simulink model "SF011A_EotLrng"  (R2013b)
settings: Solver=FixedStepDiscrete  SolverMode=SingleTasking  StartTime=0.0  StopTime=1  FixedStep=0.002  RelTol=1e-3
values from neighbouring files (symbols this model uses):
  ARCHGLBPRM_FLOATZEROTHD_ULS_F32 = DataDict.Constant    [SF011A_EotLrng_DataDict.m]
  CNVTOMILLISEC_MILLISECPERCNT_F32 = DataDict.Constant    [SF011A_EotLrng_DataDict.m]
  CORRLNFLT_CNT_U08 = DataDict.Constant    [SF011A_EotLrng_DataDict.m]
  DEBSTEP_CNT_U16 = DataDict.Constant    [SF011A_EotLrng_DataDict.m]
  EOTLIMDETD_CNT_LOGL = DataDict.Constant    [SF011A_EotLrng_DataDict.m]
  EOTLIMNOTDETD_CNT_LOGL = DataDict.Constant    [SF011A_EotLrng_DataDict.m]
  EotLrngAuthyStrtLrn = DataDict.Calibration    [SF011A_EotLrng_DataDict.m]
  EotLrngEotLrnTmr = DataDict.Calibration    [SF011A_EotLrng_DataDict.m]
  EotLrngHwAgOverTrvlCnt = DataDict.Calibration    [SF011A_EotLrng_DataDict.m]
  EotLrngHwAgOverTrvlEntr = DataDict.Calibration    [SF011A_EotLrng_DataDict.m]
  EotLrngHwAgOverTrvlExit = DataDict.Calibration    [SF011A_EotLrng_DataDict.m]
  EotLrngHwTqEotLrn = DataDict.Calibration    [SF011A_EotLrng_DataDict.m]
  EotLrngMotVelEotLrn = DataDict.Calibration    [SF011A_EotLrng_DataDict.m]
  EotLrngRackTrvlMax = DataDict.Calibration    [SF011A_EotLrng_DataDict.m]
  EotLrngRackTrvlMin = DataDict.Calibration    [SF011A_EotLrng_DataDict.m]
  EotLrngRstAuthyMin = DataDict.Calibration    [SF011A_EotLrng_DataDict.m]
  EotProtnRackTrvlLimrEna = DataDict.ImprtdCal    [SF011A_EotLrng_DataDict.m]
  HwAgOverTrvl = DataDict.NTC    [SF011A_EotLrng_DataDict.m]
  HWAGOVERTRVLMAXCNT_CNT_U08 = DataDict.Constant    [SF011A_EotLrng_DataDict.m]
  NODEBSTEP_CNT_U16 = DataDict.Constant    [SF011A_EotLrng_DataDict.m]
  OUTOFRNGFLT_CNT_U08 = DataDict.Constant    [SF011A_EotLrng_DataDict.m]
  RackEotStorgFlt = DataDict.NTC    [SF011A_EotLrng_DataDict.m]
  SIGAVLFLT_CNT_U08 = DataDict.Constant    [SF011A_EotLrng_DataDict.m]
undefined symbols (not defined in the file or in its folder): NtcSts1, NvmGetErrSts1, SigQlfr1
libraries: simulink x19, NxtrNvM x12, NxtrAbslt x5, NxtrLim x4, NxtrMax x3, NxtrMin x3
(part 1 of 7)
Description:
  | This function uses vehicle operational information to learn the appropriate end of travel positions for a given system.  Since the position end stop information is important for such functions as
  | end of travel protection to mechanically protect the gear and since the data can vary from one system to the next, it is important to learn these positions
  | 
  | The design also includes features to allow learning to reactivate under conditions of failure or diaganostic service requests (e.g. alignment).
settings Model: PauseTimes=0.35  CovFilter=UTP_SF011A_EotLrng_cov_flt_list  CovHTMLOptions=-sRT=1 -aTS=1 -bRG=1 -bTC=1 -hTR=0 -nFC=0 -scm=1 -bcm=1 -xEv=0  Creator=Mark Kushion  LastModifiedBy=NZ2988
settings SolverCC: AutoInsertRateTranBlk=on  InsertRTBMode=Always
settings DataIOCC: LimitDataPoints=off  SaveFormat=Structure  ReturnWorkspaceOutputs=on
settings OptimizationCC: BlockReduction=off  InlineParams=on  ZeroExternalMemoryAtStartup=off  ZeroInternalMemoryAtStartup=off  OptimizeModelRefInitCode=on  LifeSpan=1
settings DebuggingCC: SignalInfNanChecking=error  SignalRangeChecking=warning  UnderspecifiedInitializationDetection=Simplified  SolverPrmCheckMsg=error  InheritedTsInSrcMsg=error  DiscreteInheritContinuousMsg=error  SingleTaskRateTransMsg=error  TasksWithSamePriorityMsg=error  SigSpecEnsureSampleTimeMsg=error  CheckMatrixSingularityMsg=error  ParameterUnderflowMsg=error  ParameterPrecisionLossMsg=error  ParameterTunabilityLossMsg=error  FixptConstUnderflowMsg=warning  FixptConstOverflowMsg=warning  VectorMatrixConversionMsg=error  SignalLabelMismatchMsg=error  UnconnectedInputMsg=error  UnconnectedOutputMsg=error  UnconnectedLineMsg=error  SFcnCompatibilityMsg=error  UniqueDataStoreMsg=warning  BusObjectLabelMismatch=error  RootOutportRequireBusObject=error  AssertControl=DisableAll  ModelReferenceIOMsg=error  ModelReferenceVersionMismatchMessage=warning  ModelReferenceIOMismatchMessage=error  ModelReferenceCSMismatchMessage=warning  ModelReferenceDataLoggingMessage=error  StateNameClashWarn=warning  StrictBusMsg=ErrorOnBusTreatedAsVector  NonBusSignalsTreatedAsBus=error  SFUnexpectedBacktrackingDiag=error  SFInvalidInputDataAccessInChartInitDiag=error  SFNoUnconditionalDefaultTransitionDiag=error  SFTransitionOutsideNaturalParentDiag=error  SFUnconditionalTransitionShadowingDiag=error  SFUndirectedBroadcastEventsDiag=error
settings ModelReferenceCC: ModelReferenceNumInstancesAllowed=Single
settings RTWCC: SystemTargetFile=autosar.tlc  GenCodeOnly=on  TemplateMakefile=ert_default_tmf  Description=AUTOSAR  GenerateReport=on  ProcessScript=autosar_make_rtw_hook  LaunchReport=on
settings CodeAppCC: GenerateComments=off  IgnoreCustomStorageClasses=off  CustomSymbolStrType=$N$R$M  CustomSymbolStrBlkIO=$N$M  SimulinkBlockComments=off
settings STFCustomTargetCC: ParMdlRefBuildCompliant=on  CompOptLevelCompliant=on  IncludeMdlTerminateFcn=off  CombineOutputUpdateFcns=on  SuppressErrorStatus=on  ERTFirstTimeCompliant=on  ERTCustomFileBanners=on  SupportNonFinite=off  SupportComplex=off  SupportContinuousTime=off  SupportNonInlinedSFcns=off  MATLABClassNameForMDSCustomization=Simulink.SoftwareTarget.ERTCustomization  AutosarCompliant=on  GRTInterface=off  SystemTargetFile=autosar.tlc
settings ERTTargetCC: CodeReplacementLibrary=ANSI_C  ConcurrentExecutionCompliant=off  IncludeMdlTerminateFcn=off  SuppressErrorStatus=on  SupportNonFinite=off  SupportComplex=off  ModelStepFunctionPrototypeControlCompliant=off  CPPClassGenCompliant=off  AutosarCompliant=on  InlinedParameterPlacement=NonHierarchical  ERTCustomFileTemplate=example_file_process.tlc  EnableUserReplacementTypes=on

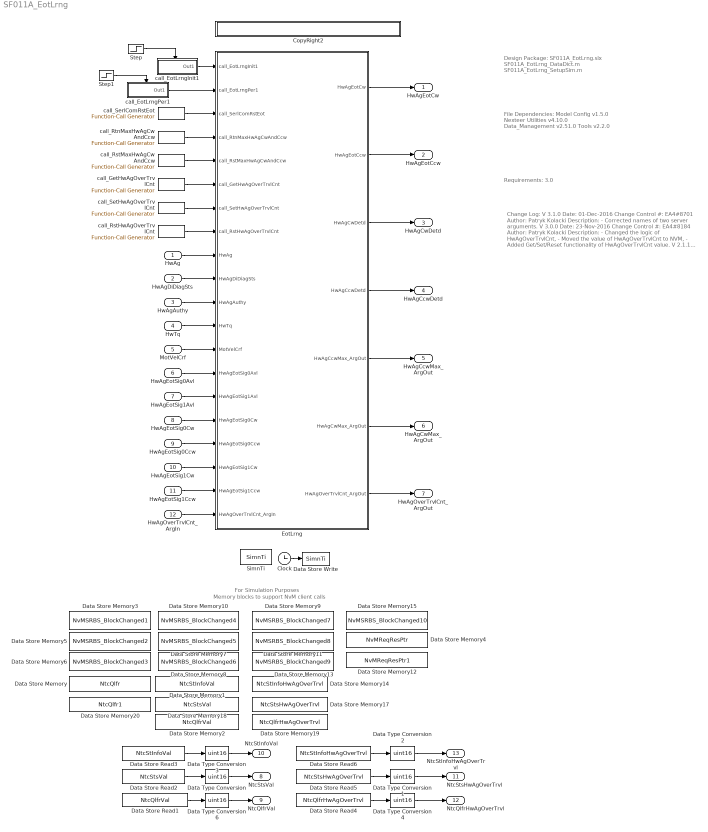
== system SF011A_EotLrng ==
  note: Requirements: 3.0
  note: File Dependencies:
      |
      | Model Config v1.5.0
      | Nexteer Utilities v4.10.0
      | Data_Management v2.51.0
      | Tools v2.2.0
  note: Change Log:
      | V 3.1.0
      | Date: 01-Dec-2016
      | Change Control #: EA4#8701
      | Author: Patryk Kolacki
      | Description:
      | - Corrected names of two server arguments.
      |
      | V 3.0.0
      | Date: 23-Nov-2016
      | Change Control #: EA4#8184
      | Author: Patryk Kolacki
      | Description:
      | - Changed the logic of HwAgOverTrvlCnt,
      | - Moved the value of HwAgOverTrvlCnt to NVM,
      | - Added Get/Set/Reset functionality of HwAgOverTrvlCnt value.
      |
      | V 2.1.1
      | Date: 02-Aug-2016
      | Change Control #: EA4#6725
      | Description:
      | - Changed the NtcQlfr to NtcQlfr1 in NTC blocks of NTC 0x0A7 for simulation
      |   purpose.
      |
      | V 2.1.0
      | Date: 13-Jun-2016
      | Change Control #: EA4#6115
      | Author: Sudeep shankar
      | Description:
      | - "Over travel" diagnostic NTC is set when HW position is outside
      | of  EOT limit.
      | - NTCNR_0X0E1.NtcTyp is changed from 'None' to 'Deb' in
      | DataDictionary for NTCNR_0X0E1 NTC.
      |
      | V 2.0.0
      | Date: 18-May-2016
      | Change Control #: EA4#5532
      | Author: Sudeep shankar
      | Description:
      | - Added logic to determine Max HwAg Cw and Ccw seen by the gear
      | over life of gear
      |
      | V 1.4.0
      | Date: 04-Jan-2016
      | Change Control #: 3583
      | Author: Shailesh Singh/Muragesh(KPIT)
      | Description:
      | - EotNvmData.EngInit changed from struct to []
      | Changed Data Store Memory 7 / Signal Attributes / Initial Value
      | from struct to []
      |
      | V 1.3.0
      | Date: 1-Oct-2015
      | Change Control #: 1216
      | Author: Sudeep Shankar
      | Description:
      | - Nvm and GetRefTmr100MicroSec32bit "Call-Location" updated in DD
      | - RTE write calls for output signals updated in DD
      | - RTE output names for Init1 are aligned with periodic
      | - Added limit blocks in Init to limit outputs
      |
      | V 1.2.0
      | Date: 28-Sep-2015
      | Change Control #: 1216
      | Author: Sudeep Shankar
      | Description:
      | - GetError Status is compared against enum to verify validity of NVM
      | - Init block is added with Min max range check of Eot limits and invoke
      |   reset Eot if out of range
      | - In periodic, Reset Eot block is replaced with the same as used in Init
      |    and updated annotation
      | - Boolean Constant name changed from '_LGC' to '_LOGL' as per
      |   EA4 naming standards
      | - Min Max range check corrected for Ccw inside SRL enable block
      |
      |
      | V1.1.0:
      | Date: 20-Sep-2105
      | Change Control #: 1216
      | Author: Sudeep Shankar
      | Description: Cw and Ccw range update in DataDictonary.
      |
      |
      | V 1.0.0
      | Date: 15-Sep-2015
      | Change Control #: 1216
      | Author: Sudeep Shankar
      | Description:
      | - Initial Release based on EA3 V 6.0.0 and added logic to use learned
      |  limits from control module based on SRL enable.
  note: For Simulation Purposes
  note: Memory blocks to support NvM client calls
  note: Design Package:
      |
      | SF011A_EotLrng.slx
      | SF011A_EotLrng_DataDict.m
      | SF011A_EotLrng_SetupSim.m
  HwAg : Inport
  HwAgDiDiagSts : Inport  Port=2
  HwAgAuthy : Inport  Port=3
  HwTq : Inport  Port=4
  MotVelCrf : Inport  Port=5
  HwAgEotSig0Avl : Inport  RequirementInfo={} %GIDa_73aa7372_5f3f_4a20_9c9f_25262da9d972  Port=6
  HwAgEotSig1Avl : Inport  RequirementInfo={} %GIDa_66c51ce2_8578_4348_9fad_52cccaaeb985  Port=7
  HwAgEotSig0Cw : Inport  RequirementInfo={} %GIDa_a5f7fcd9_8a24_4cbe_b701_71991071193b  Port=8
  HwAgEotSig0Ccw : Inport  RequirementInfo={} %GIDa_9a8ac91a_a1c0_4442_a2c5_4b419678d76d  Port=9
  HwAgEotSig1Cw : Inport  RequirementInfo={} %GIDa_8f8e183e_8cba_4267_90ea_415514e5b391  Port=10
  HwAgEotSig1Ccw : Inport  RequirementInfo={} %GIDa_19e35c30_ed39_4f4a_8321_5e5ce81c406e  Port=11
  HwAgOverTrvlCnt_ArgIn : Inport  RequirementInfo={} %GIDa_de79dbd8_1f60_4db4_9d0d_a8f19dcbcdc4  Port=12
  Clock : Clock
  CopyRight2 : Subsystem  Description=|  mask(Copyright Information){none=on}
      | Copyright info block.                                               
      |                                                                     
      | Place copyright information at the top of every subsystem in design.
      mask prompts: none "No parameters"
      mask help: Place copyright information at the top of every subsystem in design.
      mask Display:
      | NxtrConf = 'Nexteer Confidential';
      | 
      | sys = bdroot; %handle for the current model ("system")
      | first = get_param(sys,'Created');
      | if(isempty(first))
      |     first = datestr(now,'yyyy');
      | else
      |     first = first(end-3:end);  %year is last four digits
      | end
      | 
      | last = get_param(sys,'LastModifiedDate');
      | if isempty(last)
      |     last = datestr(now,'yyyy');
      | else
      |     last = last(end-3:end);
      | end
      | 
      | if strcmp(first,last)
      |     fprintf('%s -- Copyright %s Nexteer',NxtrConf,first)
      | else
      |     fprintf('%s -- %s%s- %s Nexteer',NxtrConf,char(169),first,last)
      | end
  Data Store Memory : DataStoreMemory  DataStoreName=NtcQlfr  InitialValue=SigQlfr1.SIGQLFR_NORES  OutDataTypeStr=Enum: SigQlfr1
  Data Store Memory1 : DataStoreMemory  DataStoreName=NtcStInfoVal  OutDataTypeStr=uint8
  Data Store Memory10 : DataStoreMemory  DataStoreName=NvMSRBS_BlockChanged4  ReadBeforeWriteMsg=warning  WriteAfterWriteMsg=warning  WriteAfterReadMsg=warning
  Data Store Memory11 : DataStoreMemory  DataStoreName=NvMSRBS_BlockChanged8  ReadBeforeWriteMsg=warning  WriteAfterWriteMsg=warning  WriteAfterReadMsg=warning
  Data Store Memory12 : DataStoreMemory  DataStoreName=NvMReqResPtr1
  Data Store Memory13 : DataStoreMemory  DataStoreName=NvMSRBS_BlockChanged9  ReadBeforeWriteMsg=warning  WriteAfterWriteMsg=warning  WriteAfterReadMsg=warning
  Data Store Memory14 : DataStoreMemory  DataStoreName=NtcStInfoHwAgOverTrvl  OutDataTypeStr=uint8
  Data Store Memory15 : DataStoreMemory  DataStoreName=NvMSRBS_BlockChanged10  ReadBeforeWriteMsg=warning  WriteAfterWriteMsg=warning  WriteAfterReadMsg=warning
  Data Store Memory17 : DataStoreMemory  DataStoreName=NtcStsHwAgOverTrvl  InitialValue=NtcSts1.NTCSTS_PASSD  OutDataTypeStr=Enum: NtcSts1
  Data Store Memory18 : DataStoreMemory  DataStoreName=NtcStsVal  InitialValue=NtcSts1.NTCSTS_PASSD  OutDataTypeStr=Enum: NtcSts1
  Data Store Memory19 : DataStoreMemory  DataStoreName=NtcQlfrHwAgOverTrvl  InitialValue=SigQlfr1.SIGQLFR_NORES  OutDataTypeStr=Enum: SigQlfr1
  Data Store Memory2 : DataStoreMemory  DataStoreName=NtcQlfrVal  InitialValue=SigQlfr1.SIGQLFR_NORES  OutDataTypeStr=Enum: SigQlfr1
  Data Store Memory20 : DataStoreMemory  DataStoreName=NtcQlfr1  InitialValue=SigQlfr1.SIGQLFR_NORES  OutDataTypeStr=Enum: SigQlfr1
  Data Store Memory3 : DataStoreMemory  DataStoreName=NvMSRBS_BlockChanged1  ReadBeforeWriteMsg=warning  WriteAfterWriteMsg=warning  WriteAfterReadMsg=warning
  Data Store Memory4 : DataStoreMemory  DataStoreName=NvMReqResPtr
  Data Store Memory5 : DataStoreMemory  DataStoreName=NvMSRBS_BlockChanged2  ReadBeforeWriteMsg=warning  WriteAfterWriteMsg=warning  WriteAfterReadMsg=warning
  Data Store Memory6 : DataStoreMemory  DataStoreName=NvMSRBS_BlockChanged3  ReadBeforeWriteMsg=warning  WriteAfterWriteMsg=warning  WriteAfterReadMsg=warning
  Data Store Memory7 : DataStoreMemory  DataStoreName=NvMSRBS_BlockChanged5  ReadBeforeWriteMsg=warning  WriteAfterWriteMsg=warning  WriteAfterReadMsg=warning
  Data Store Memory8 : DataStoreMemory  DataStoreName=NvMSRBS_BlockChanged6  ReadBeforeWriteMsg=warning  WriteAfterWriteMsg=warning  WriteAfterReadMsg=warning
  Data Store Memory9 : DataStoreMemory  DataStoreName=NvMSRBS_BlockChanged7  ReadBeforeWriteMsg=warning  WriteAfterWriteMsg=warning  WriteAfterReadMsg=warning
  Data Store Read1 : DataStoreRead  DataStoreName=NtcQlfrVal  SampleTime=.010
  Data Store Read2 : DataStoreRead  DataStoreName=NtcStsVal  SampleTime=.010
  Data Store Read3 : DataStoreRead  DataStoreName=NtcStInfoVal  SampleTime=.010
  Data Store Read4 : DataStoreRead  DataStoreName=NtcQlfrHwAgOverTrvl  SampleTime=.010
  Data Store Read5 : DataStoreRead  DataStoreName=NtcStsHwAgOverTrvl  SampleTime=.010
  Data Store Read6 : DataStoreRead  DataStoreName=NtcStInfoHwAgOverTrvl  SampleTime=.010
  Data Store Write : DataStoreWrite  DataStoreName=SimnTi
  Data Type Conversion{,1..4,6} (6 alike) : DataTypeConversion  OutDataTypeStr=uint16
  EotLrng : Subsystem
  SimnTi : DataStoreMemory  DataStoreName=SimnTi
  Step : Step  Time=.001  Before=1  After=0  SampleTime=0
  Step1 : Step  Time=.001  SampleTime=0
  call_EotLrngInit1 : Subsystem  TreatAsAtomicUnit=on
  call_EotLrngPer1 : Subsystem  TreatAsAtomicUnit=on
  call_GetHwAgOverTrvlCnt : simulink/Ports & Subsystems/Function-Call Generator  RequirementInfo={} %GIDa_e3baf494_81de_4b12_b72d_b79894e06156  sample_time=0.010  numberOfIterations=1
  call_RstHwAgOverTrvlCnt : simulink/Ports & Subsystems/Function-Call Generator  RequirementInfo={} %GIDa_03bc3f2a_ba1d_4971_9b17_2c952515d504  sample_time=0.010  numberOfIterations=1
  call_RstMaxHwAgCwAndCcw : simulink/Ports & Subsystems/Function-Call Generator  RequirementInfo={} %GIDa_ce2e9b2d_63af_495d_a1f3_e9201e666fa9  sample_time=0.010  numberOfIterations=1
  call_RtnMaxHwAgCwAndCcw : simulink/Ports & Subsystems/Function-Call Generator  RequirementInfo={} %GIDa_042fcac4_2799_4e4f_8586_b1f6181d77cc  sample_time=0.010  numberOfIterations=1
  call_SerlComRstEot : simulink/Ports & Subsystems/Function-Call Generator  RequirementInfo={} %GIDa_78894832_b76f_4101_86f3_f5347d110ee9  sample_time=0.010  numberOfIterations=1
  call_SetHwAgOverTrvlCnt : simulink/Ports & Subsystems/Function-Call Generator  RequirementInfo={} %GIDa_ec1b0ef1_ec8f_4026_a564_0387bacc0f1d  sample_time=0.010  numberOfIterations=1
  HwAgEotCw : Outport
  HwAgEotCcw : Outport  Port=2
  HwAgCwDetd : Outport  Port=3
  HwAgCcwDetd : Outport  Port=4
  HwAgCcwMax_ArgOut : Outport  Port=5
  HwAgCwMax_ArgOut : Outport  Port=6
  HwAgOverTrvlCnt_ArgOut : Outport  Port=7
  NtcStsVal : Outport  Port=8
  NtcQlfrVal : Outport  Port=9
  NtcStInfoVal : Outport  Port=10
  NtcStsHwAgOverTrvl : Outport  Port=11
  NtcQlfrHwAgOverTrvl : Outport  Port=12
  NtcStInfoHwAgOverTrvl : Outport  Port=13
  wires:
  Clock/1 -> Data Store Write/1
  EotLrng/3(HwAgCwDetd) -> HwAgCwDetd/1
  EotLrng/2(HwAgEotCcw) -> HwAgEotCcw/1
  EotLrng/1(HwAgEotCw) -> HwAgEotCw/1
  EotLrng/4(HwAgCcwDetd) -> HwAgCcwDetd/1
  call_EotLrngInit1/1(Out1) -> EotLrng/1(call_EotLrngInit1)
  Step/1 -> call_EotLrngInit1/Enable
  Step1/1 -> call_EotLrngPer1/Enable
  call_EotLrngPer1/1(Out1) -> EotLrng/2(call_EotLrngPer1)
  call_SerlComRstEot/1 -> EotLrng/3(call_SerlComRstEot)
  Data Store Read1/1 -> Data Type Conversion6/1
  Data Store Read2/1 -> Data Type Conversion/1
  Data Store Read3/1 -> Data Type Conversion3/1
  call_RtnMaxHwAgCwAndCcw/1 -> EotLrng/4(call_RtnMaxHwAgCwAndCcw)
  EotLrng/5(HwAgCcwMax_ArgOut) -> HwAgCcwMax_ArgOut/1
  EotLrng/6(HwAgCwMax_ArgOut) -> HwAgCwMax_ArgOut/1
  call_RstMaxHwAgCwAndCcw/1 -> EotLrng/5(call_RstMaxHwAgCwAndCcw)
  Data Store Read4/1 -> Data Type Conversion4/1
  Data Store Read5/1 -> Data Type Conversion1/1
  Data Store Read6/1 -> Data Type Conversion2/1
  Data Type Conversion2/1 -> NtcStInfoHwAgOverTrvl/1
  Data Type Conversion4/1 -> NtcQlfrHwAgOverTrvl/1
  Data Type Conversion1/1 -> NtcStsHwAgOverTrvl/1
  Data Type Conversion3/1 -> NtcStInfoVal/1
  Data Type Conversion6/1 -> NtcQlfrVal/1
  Data Type Conversion/1 -> NtcStsVal/1
  EotLrng/7(HwAgOverTrvlCnt_ArgOut) -> HwAgOverTrvlCnt_ArgOut/1
  call_GetHwAgOverTrvlCnt/1 -> EotLrng/6(call_GetHwAgOverTrvlCnt)
  call_SetHwAgOverTrvlCnt/1 -> EotLrng/7(call_SetHwAgOverTrvlCnt)
  call_RstHwAgOverTrvlCnt/1 -> EotLrng/8(call_RstHwAgOverTrvlCnt)
  HwAg/1 -> EotLrng/9(HwAg)
  HwAgDiDiagSts/1 -> EotLrng/10(HwAgDiDiagSts)
  HwAgAuthy/1 -> EotLrng/11(HwAgAuthy)
  HwTq/1 -> EotLrng/12(HwTq)
  MotVelCrf/1 -> EotLrng/13(MotVelCrf)
  HwAgEotSig0Avl/1 -> EotLrng/14(HwAgEotSig0Avl)
  HwAgOverTrvlCnt_ArgIn/1 -> EotLrng/20(HwAgOverTrvlCnt_ArgIn)
  HwAgEotSig1Ccw/1 -> EotLrng/19(HwAgEotSig1Ccw)
  HwAgEotSig1Cw/1 -> EotLrng/18(HwAgEotSig1Cw)
  HwAgEotSig0Ccw/1 -> EotLrng/17(HwAgEotSig0Ccw)
  HwAgEotSig0Cw/1 -> EotLrng/16(HwAgEotSig0Cw)
  HwAgEotSig1Avl/1 -> EotLrng/15(HwAgEotSig1Avl)

== system SF011A_EotLrng/CopyRight2 ==

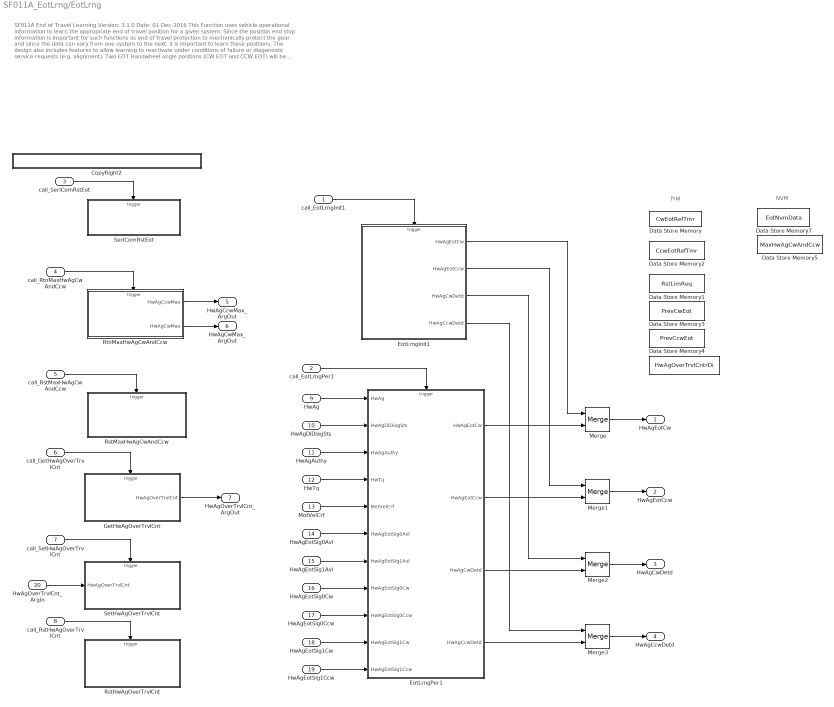
== system SF011A_EotLrng/EotLrng ==
  note: NVM
  note: PIM
  note: SF011A              End of Travel Learning            Version: 3.1.0         Date: 01-Dec-2016
      |
      | This Function uses vehicle operational information to learn the appropriate end of travel position for a given system. Since the position end stop information
      | is important for such functions as end of travel protection to mechanically protect the gear and since the data can vary from one system to the next, it is
      | important to learn these positions.
      |
      | The design also includes features to allow learning to reactivate under conditions of failure or diaganostic service requests (e.g. alignment).
      |
      |  Two EOT Handwheel angle positions (CW EOT and CCW EOT) will be stored in the scratchpad of HW Torque Sensor 0 with a redundant copy  also stored
      |  in the scratchpad of HW Torque Sensor 1 during manufacturing build up. These CW and CCW EOT values will be used for providing the Software Rack
      |  Travel Limits when EotProtnRackTrvlLimrEna is True.
  call_EotLrngInit1 : Inport
  call_EotLrngPer1 : Inport  Port=2
  call_SerlComRstEot : Inport  Port=3
  call_RtnMaxHwAgCwAndCcw : Inport  Port=4
  call_RstMaxHwAgCwAndCcw : Inport  Port=5
  call_GetHwAgOverTrvlCnt : Inport  RequirementInfo={} %GIDa_1cc9e590_aebc_4faa_bf48_c1a914c9f56c  Port=6
  call_SetHwAgOverTrvlCnt : Inport  RequirementInfo={} %GIDa_33957908_3297_46c1_8714_52d5541ebe06  Port=7
  call_RstHwAgOverTrvlCnt : Inport  RequirementInfo={} %GIDa_b35ca6d8_d86b_4ebc_a4ac_db0bdb5da668  Port=8
  HwAg : Inport  RequirementInfo="{'linktype_rmi_doors' '0000ba59 (/E-STEER Core/SubSystem Specifications/Application Functions/SF011A Learned EOT Limits)' '#SF011A_9' 'true' 'REQ:  SF011A_9' '' } %GIDa_42db33ca_01d7_41c2_af64_efb098aee0cd"  Port=9
  HwAgDiDiagSts : Inport  RequirementInfo="{'linktype_rmi_doors' '0000ba59 (/E-STEER Core/SubSystem Specifications/Application Functions/SF011A Learned EOT Limits)' '#SF011A_36' 'true' 'REQ:  SF011A_36' '' } %GIDa_ec3a5a8a_8e2b_48db_b047_1f602cc7cc9a"  Port=10
  HwAgAuthy : Inport  RequirementInfo="{'linktype_rmi_doors' '0000ba59 (/E-STEER Core/SubSystem Specifications/Application Functions/SF011A Learned EOT Limits)' '#SF011A_32' 'true' 'REQ:  SF011A_32' '' } %GIDa_27f0f5a0_b684_4830_bfd2_ef6d05a05c0b"  Port=11
  HwTq : Inport  RequirementInfo="{'linktype_rmi_doors' '0000ba59 (/E-STEER Core/SubSystem Specifications/Application Functions/SF011A Learned EOT Limits)' '#SF011A_34' 'true' 'REQ:  SF011A_34' '' } %GIDa_8b7c6650_fd63_4843_9db1_7f1e52f08757"  Port=12
  MotVelCrf : Inport  RequirementInfo="{'linktype_rmi_doors' '0000ba59 (/E-STEER Core/SubSystem Specifications/Application Functions/SF011A Learned EOT Limits)' '#SF011A_33' 'true' 'REQ:  SF011A_33' '' } %GIDa_72ce3fd6_9cc5_4395_adf3_db347db2b3a0"  Port=13
  HwAgEotSig0Avl : Inport  RequirementInfo="{'linktype_rmi_doors' '0000ba59 (/E-STEER Core/SubSystem Specifications/Application Functions/SF011A Learned EOT Limits)' '#SF011A_116' 'true' 'REQ:  SF011A_116' '' } %GIDa_80459358_5b4f_48e6_a7b8_8da9c9038f81"  Port=14
  HwAgEotSig1Avl : Inport  RequirementInfo="{'linktype_rmi_doors' '0000ba59 (/E-STEER Core/SubSystem Specifications/Application Functions/SF011A Learned EOT Limits)' '#SF011A_116' 'true' 'REQ:  SF011A_116' '' } %GIDa_3caee551_e75b_4d25_be80_97aaac300dbd"  Port=15
  HwAgEotSig0Cw : Inport  RequirementInfo="{'linktype_rmi_doors' '0000ba59 (/E-STEER Core/SubSystem Specifications/Application Functions/SF011A Learned EOT Limits)' '#SF011A_117' 'true' 'REQ:  SF011A_117' '' } %GIDa_c15a533c_6152_4a8a_b933_7aad34b2e7de"  Port=16
  HwAgEotSig0Ccw : Inport  RequirementInfo="{'linktype_rmi_doors' '0000ba59 (/E-STEER Core/SubSystem Specifications/Application Functions/SF011A Learned EOT Limits)' '#SF011A_118' 'true' 'REQ:  SF011A_118' '' } %GIDa_4930c781_ec4f_4ebe_87d2_655a305eb055"  Port=17
  HwAgEotSig1Cw : Inport  RequirementInfo="{'linktype_rmi_doors' '0000ba59 (/E-STEER Core/SubSystem Specifications/Application Functions/SF011A Learned EOT Limits)' '#SF011A_117' 'true' 'REQ:  SF011A_117' '' } %GIDa_5965b097_97b2_4555_a032_94a0a70ed026"  Port=18
  HwAgEotSig1Ccw : Inport  RequirementInfo="{'linktype_rmi_doors' '0000ba59 (/E-STEER Core/SubSystem Specifications/Application Functions/SF011A Learned EOT Limits)' '#SF011A_118' 'true' 'REQ:  SF011A_118' '' } %GIDa_7afbb674_d8de_4557_8f9d_4901633a5dc2"  Port=19
  HwAgOverTrvlCnt_ArgIn : Inport  RequirementInfo="{'linktype_rmi_doors' '0000ba59 (/E-STEER Core/SubSystem Specifications/Application Functions/SF011A Learned EOT Limits)' '#SF011A_201' 'true' 'REQ:  SF011A_201' '' } %GIDa_bf5dc2c4_d885_475e_9768_988ed04b3a3b"  Port=20
  " " : DataStoreMemory  DataStoreName=HwAgOverTrvlCntrDi  StateMustResolveToSignalObject=on
  CopyRight2 : Subsystem  Description=|  mask(Copyright Information){none=on}
      | Copyright info block.                                               
      |                                                                     
      | Place copyright information at the top of every subsystem in design.
      mask prompts: none "No parameters"
      mask help: Place copyright information at the top of every subsystem in design.
      mask Display:
      | NxtrConf = 'Nexteer Confidential';
      | 
      | sys = bdroot; %handle for the current model ("system")
      | first = get_param(sys,'Created');
      | if(isempty(first))
      |     first = datestr(now,'yyyy');
      | else
      |     first = first(end-3:end);  %year is last four digits
      | end
      | 
      | last = get_param(sys,'LastModifiedDate');
      | if isempty(last)
      |     last = datestr(now,'yyyy');
      | else
      |     last = last(end-3:end);
      | end
      | 
      | if strcmp(first,last)
      |     fprintf('%s -- Copyright %s Nexteer',NxtrConf,first)
      | else
      |     fprintf('%s -- %s%s- %s Nexteer',NxtrConf,char(169),first,last)
      | end
  Data Store Memory : DataStoreMemory  DataStoreName=CwEotRefTmr  StateMustResolveToSignalObject=on
  Data Store Memory1 : DataStoreMemory  DataStoreName=RstLimReq  StateMustResolveToSignalObject=on
  Data Store Memory2 : DataStoreMemory  DataStoreName=CcwEotRefTmr  StateMustResolveToSignalObject=on
  Data Store Memory3 : DataStoreMemory  DataStoreName=PrevCwEot  StateMustResolveToSignalObject=on
  Data Store Memory4 : DataStoreMemory  DataStoreName=PrevCcwEot  StateMustResolveToSignalObject=on
  Data Store Memory5 : DataStoreMemory  RequirementInfo="{'linktype_rmi_doors' '0000ba59 (/E-STEER Core/SubSystem Specifications/Application Functions/SF011A Learned EOT Limits)' '#SF011A_209' 'true' 'REQ:  SF011A_209' '' } %GIDa_e44e0bfb_d806_48d4_a199_844757409d5d"  DataStoreName=MaxHwAgCwAndCcw  InitialValue=[]  OutDataTypeStr=Bus: MaxHwAgCwAndCcwRec2  StateMustResolveToSignalObject=on
  Data Store Memory7 : DataStoreMemory  RequirementInfo="{'linktype_rmi_doors' '0000ba59 (/E-STEER Core/SubSystem Specifications/Application Functions/SF011A Learned EOT Limits)' '#SF011A_59' 'true' 'REQ:  SF011A_59' '' ; 'linktype_rmi_doors' '0000ba59 (/E-STEER Core/SubSystem Specifications/Application Functions/SF011A Learned EOT Limits)' '#SF011A_63' 'true' 'REQ:  SF011A_63' '' ; 'linktype_rmi_doors' '0000ba59 (/E-STEER Core/SubSystem Specifications/Application Functions/SF011A Learned EOT Limits)' '#SF011A_62' 'true' 'REQ:  SF011A_62' '' ; 'linktype_rmi_doors' '0000ba59 (/E-STEER Core/SubSystem Specifications/Application Functions/SF011A Learned EOT Limits)' '#SF011A_61' 'true' 'REQ:  SF011A_61' '' ; 'linktype_rmi_doors' '0000ba59 (/E-STEER Core/SubSystem Specifications/Application Functions/SF011A Learned EOT Limits)' '#SF011A_60' 'true' 'REQ:  SF011A_60' '' ; 'linktype_rmi_doors' '0000ba59 (/E-STEER Core/SubSystem Specifications/Application Functions/SF011A Learned EOT Limits)' '#SF011A_111' 'true' 'REQ:  SF011A_111' '' ; 'linktype_rmi_doors' '0000ba59 (/E-STEER Core/SubSystem Specifications/Application Functions/SF011A Learned EOT Limits)' '#SF011A_112' 'true' 'REQ:  SF011A_112' '' ; 'linktype_rmi_doors' '0000ba59 (/E-STEER Core/SubSystem Specifications/Application Functions/SF011A Learned EOT Limits)' '#SF011A_113' 'true' 'REQ:  SF011A_113' '' ; 'linktype_rmi_doors' '0000ba59 (/E-STEER Core/SubSystem Specifications/Application Functions/SF011A Learned EOT Limits)' '#SF011A_114' 'true' 'REQ:  SF011A_114' '' } %GIDa_e5eb2182_a554_401e_b57f_80817cd7d6f2"  DataStoreName=EotNvmData  InitialValue=[]  OutDataTypeStr=Bus: EotNvmDataRec1  StateMustResolveToSignalObject=on
  EotLrngInit1 : Subsystem
  EotLrngPer1 : Subsystem
  GetHwAgOverTrvlCnt : Subsystem  RequirementInfo="{'linktype_rmi_doors' '0000ba59 (/E-STEER Core/SubSystem Specifications/Application Functions/SF011A Learned EOT Limits)' '#SF011A_203' 'true' 'REQ:  SF011A_203' '' } %GIDa_4a5e5f15_a9c8_48fe_986b_cbf465310d0d"
  Merge{,1..3} (4 alike) : Merge
  RstHwAgOverTrvlCnt : Subsystem  RequirementInfo="{'linktype_rmi_doors' '0000ba59 (/E-STEER Core/SubSystem Specifications/Application Functions/SF011A Learned EOT Limits)' '#SF011A_195' 'true' 'REQ:  SF011A_195' '' } %GIDa_9394070d_1ce8_4ba7_93f9_e1140329ccb6"
  RstMaxHwAgCwAndCcw : Subsystem  RequirementInfo="{'linktype_rmi_doors' '0000ba59 (/E-STEER Core/SubSystem Specifications/Application Functions/SF011A Learned EOT Limits)' '#SF011A_160' 'true' 'REQ:  SF011A_160' '' } %GIDa_1fbc0f2a_c98c_4700_a26d_603b800c132e"
  RtnMaxHwAgCwAndCcw : Subsystem  RequirementInfo="{'linktype_rmi_doors' '0000ba59 (/E-STEER Core/SubSystem Specifications/Application Functions/SF011A Learned EOT Limits)' '#SF011A_161' 'true' 'REQ:  SF011A_161' '' } %GIDa_68e311d9_bd4a_4580_880d_d3fc2cfa134d"
  SerlComRstEot : Subsystem  RequirementInfo="{'linktype_rmi_doors' '0000ba59 (/E-STEER Core/SubSystem Specifications/Application Functions/SF011A Learned EOT Limits)' '#SF011A_122' 'true' 'REQ:  SF011A_122' '' } %GIDa_2196a33e_1ec6_460e_afc4_c4580f78035f"
  SetHwAgOverTrvlCnt : Subsystem  RequirementInfo="{'linktype_rmi_doors' '0000ba59 (/E-STEER Core/SubSystem Specifications/Application Functions/SF011A Learned EOT Limits)' '#SF011A_200' 'true' 'REQ:  SF011A_200' '' } %GIDa_51ef5841_6e7a_4466_9fdc_0a858abb14eb"
  HwAgEotCw : Outport  RequirementInfo="{'linktype_rmi_doors' '0000ba59 (/E-STEER Core/SubSystem Specifications/Application Functions/SF011A Learned EOT Limits)' '#SF011A_11' 'true' 'REQ:  SF011A_11' '' } %GIDa_41bb65f1_1f75_476c_89b3_1b3c930dd361"
  HwAgEotCcw : Outport  RequirementInfo="{'linktype_rmi_doors' '0000ba59 (/E-STEER Core/SubSystem Specifications/Application Functions/SF011A Learned EOT Limits)' '#SF011A_39' 'true' 'REQ:  SF011A_39' '' } %GIDa_1bef1b8e_eaa3_4452_9aff_1fc22e093c45"  Port=2
  HwAgCwDetd : Outport  RequirementInfo="{'linktype_rmi_doors' '0000ba59 (/E-STEER Core/SubSystem Specifications/Application Functions/SF011A Learned EOT Limits)' '#SF011A_40' 'true' 'REQ:  SF011A_40' '' } %GIDa_78cdf14d_76bb_44d2_9d5f_dfd0819f21ed"  Port=3
  HwAgCcwDetd : Outport  RequirementInfo="{'linktype_rmi_doors' '0000ba59 (/E-STEER Core/SubSystem Specifications/Application Functions/SF011A Learned EOT Limits)' '#SF011A_41' 'true' 'REQ:  SF011A_41' '' } %GIDa_3fe008c8_2677_4027_a610_4cee2f6e870d"  Port=4
  HwAgCcwMax_ArgOut : Outport  RequirementInfo={} %GIDa_3eec765e_d5a4_4357_9ae4_04adabccafe6  Port=5
  HwAgCwMax_ArgOut : Outport  RequirementInfo={} %GIDa_2634233d_75b1_4c53_9d31_6713fad6f33b  Port=6
  HwAgOverTrvlCnt_ArgOut : Outport  RequirementInfo={} %GIDa_8619cd48_f7b1_49f8_ae7e_1504e94fcefc  Port=7
  wires:
  call_EotLrngPer1/1 -> EotLrngPer1/Trigger
  call_SerlComRstEot/1 -> SerlComRstEot/Trigger
  call_EotLrngInit1/1 -> EotLrngInit1/Trigger
  Merge3/1 -> HwAgCcwDetd/1
  EotLrngPer1/4(HwAgCcwDetd) -> Merge3/2
  EotLrngPer1/3(HwAgCwDetd) -> Merge2/2
  EotLrngPer1/2(HwAgEotCcw) -> Merge1/2
  Merge/1 -> HwAgEotCw/1
  Merge1/1 -> HwAgEotCcw/1
  Merge2/1 -> HwAgCwDetd/1
  EotLrngPer1/1(HwAgEotCw) -> Merge/2
  EotLrngInit1/1(HwAgEotCw) -> Merge/1
  EotLrngInit1/2(HwAgEotCcw) -> Merge1/1
  EotLrngInit1/3(HwAgCwDetd) -> Merge2/1
  EotLrngInit1/4(HwAgCcwDetd) -> Merge3/1
  call_RtnMaxHwAgCwAndCcw/1 -> RtnMaxHwAgCwAndCcw/Trigger
  RtnMaxHwAgCwAndCcw/1(HwAgCcwMax) -> HwAgCcwMax_ArgOut/1
  RtnMaxHwAgCwAndCcw/2(HwAgCwMax) -> HwAgCwMax_ArgOut/1
  call_RstMaxHwAgCwAndCcw/1 -> RstMaxHwAgCwAndCcw/Trigger
  GetHwAgOverTrvlCnt/1(HwAgOverTrvlCnt) -> HwAgOverTrvlCnt_ArgOut/1
  HwAgOverTrvlCnt_ArgIn/1 -> SetHwAgOverTrvlCnt/1(HwAgOverTrvlCnt)
  call_GetHwAgOverTrvlCnt/1 -> GetHwAgOverTrvlCnt/Trigger
  call_SetHwAgOverTrvlCnt/1 -> SetHwAgOverTrvlCnt/Trigger
  call_RstHwAgOverTrvlCnt/1 -> RstHwAgOverTrvlCnt/Trigger
  HwAg/1 -> EotLrngPer1/1(HwAg)
  HwAgDiDiagSts/1 -> EotLrngPer1/2(HwAgDiDiagSts)
  HwAgAuthy/1 -> EotLrngPer1/3(HwAgAuthy)
  HwTq/1 -> EotLrngPer1/4(HwTq)
  MotVelCrf/1 -> EotLrngPer1/5(MotVelCrf)
  HwAgEotSig0Avl/1 -> EotLrngPer1/6(HwAgEotSig0Avl)
  HwAgEotSig1Avl/1 -> EotLrngPer1/7(HwAgEotSig1Avl)
  HwAgEotSig0Cw/1 -> EotLrngPer1/8(HwAgEotSig0Cw)
  HwAgEotSig0Ccw/1 -> EotLrngPer1/9(HwAgEotSig0Ccw)
  HwAgEotSig1Cw/1 -> EotLrngPer1/10(HwAgEotSig1Cw)
  HwAgEotSig1Ccw/1 -> EotLrngPer1/11(HwAgEotSig1Ccw)

== system SF011A_EotLrng/call_EotLrngInit1 ==
  Enable : EnablePort
  CopyRight2 : Subsystem  Description=|  mask(Copyright Information){none=on}
      | Copyright info block.                                               
      |                                                                     
      | Place copyright information at the top of every subsystem in design.
      mask prompts: none "No parameters"
      mask help: Place copyright information at the top of every subsystem in design.
      mask Display:
      | NxtrConf = 'Nexteer Confidential';
      | 
      | sys = bdroot; %handle for the current model ("system")
      | first = get_param(sys,'Created');
      | if(isempty(first))
      |     first = datestr(now,'yyyy');
      | else
      |     first = first(end-3:end);  %year is last four digits
      | end
      | 
      | last = get_param(sys,'LastModifiedDate');
      | if isempty(last)
      |     last = datestr(now,'yyyy');
      | else
      |     last = last(end-3:end);
      | end
      | 
      | if strcmp(first,last)
      |     fprintf('%s -- Copyright %s Nexteer',NxtrConf,first)
      | else
      |     fprintf('%s -- %s%s- %s Nexteer',NxtrConf,char(169),first,last)
      | end
  Function-Call Generator : simulink/Ports & Subsystems/Function-Call Generator  sample_time=.010  numberOfIterations=1
  Out1 : Outport
  wires:
  Function-Call Generator/1 -> Out1/1

== system SF011A_EotLrng/call_EotLrngPer1 ==
  Enable : EnablePort
  CopyRight2 : Subsystem  Description=|  mask(Copyright Information){none=on}
      | Copyright info block.                                               
      |                                                                     
      | Place copyright information at the top of every subsystem in design.
      mask prompts: none "No parameters"
      mask help: Place copyright information at the top of every subsystem in design.
      mask Display:
      | NxtrConf = 'Nexteer Confidential';
      | 
      | sys = bdroot; %handle for the current model ("system")
      | first = get_param(sys,'Created');
      | if(isempty(first))
      |     first = datestr(now,'yyyy');
      | else
      |     first = first(end-3:end);  %year is last four digits
      | end
      | 
      | last = get_param(sys,'LastModifiedDate');
      | if isempty(last)
      |     last = datestr(now,'yyyy');
      | else
      |     last = last(end-3:end);
      | end
      | 
      | if strcmp(first,last)
      |     fprintf('%s -- Copyright %s Nexteer',NxtrConf,first)
      | else
      |     fprintf('%s -- %s%s- %s Nexteer',NxtrConf,char(169),first,last)
      | end
  Function-Call Generator : simulink/Ports & Subsystems/Function-Call Generator  RequirementInfo={} %GIDa_c718c7cf_dd39_4fde_b3df_6c879d412d6a  sample_time=0.010  numberOfIterations=1
  Out1 : Outport
  wires:
  Function-Call Generator/1 -> Out1/1

== system SF011A_EotLrng/EotLrng/CopyRight2 ==
